simulink library "xpcmeasurementcomputinglib"  (Simulink 6.0)
settings: Solver=ode45  SolverMode=SingleTasking  StartTime=0.0  StopTime=10.0  RelTol=1e-3
undefined symbols (not defined in the file or in its folder): madcbciodas, madcbpcidas, madcbpcidas1600, mctr05checks, mdacbisa, mdacbpcidas, mdacbpcidas1600, mdacbpcidda0x12, mdiocbpcipdisox, menccbcioquadcount, misa8255, mpci8255, mtccb
libraries: xpcmeasurementcomputinglib x18
(part 2 of 4)

== system xpcmeasurementcomputinglib/D/A ==
  "CIO-DAC08 " : S-Function  InitFcn=mdacbisa(1);  FunctionName=dacbisa  Parameters=channel, range, reset, initValue, sampletime, baseaddress, boardType  mask(dacbisa){channel=[1], range=[-10], reset=[1], initValue=[0], sampletime=0.001, baseaddress=0x300}
      mask prompts: channel "Channel vector:"; range "Range vector:"; reset "Reset vector:"; initValue "Initial value vector:"; sampletime "Sample time:"; baseaddress "Base address (i.e. 0xd000):"
      mask help:
      | CIO-DAC08
      | ComputerBoards
      | Analog Output
      mask init:
      | baseaddress=hex2dec(baseaddress(3:end));
      | boardType=2;
      | [reset, initValue] = mdacbisa(2, channel, range, reset, initValue, baseaddress, boardType);
      mask Help: helpview(fullfile(docroot, 'mapfiles', 'xpc.map'), 'ComputerBoards_CIO-DAC08_DA')
      mask Display: disp('CIO-DAC08\nComputerBoards\nAnalog Output');port_label('input',1,'1');
  "CIO-DAC08 16 " : S-Function  InitFcn=mdacbisa(1);  FunctionName=dacbisa  Parameters=channel, range, reset, initValue, sampletime, baseaddress, boardType  mask(dacbisa){channel=[1], range=[-10], reset=[1], initValue=[0], sampletime=0.001, baseaddress=0x300}
      mask prompts: channel "Channel vector:"; range "Range vector:"; reset "Reset vector:"; initValue "Initial value vector:"; sampletime "Sample time:"; baseaddress "Base address (i.e. 0xd000):"
      mask help:
      | CIO-DAC08/16
      | ComputerBoards
      | Analog Output
      mask init:
      | baseaddress=hex2dec(baseaddress(3:end));
      | boardType=5;
      | [reset, initValue] = mdacbisa(2, channel, range, reset, initValue, baseaddress, boardType);
      mask Help: helpview(fullfile(docroot, 'mapfiles', 'xpc.map'), 'ComputerBoards_CIO-DAC08-16_DA')
      mask Display: disp('CIO-DAC08/16\nComputerBoards\nAnalog Output');port_label('input',1,'1');
  "CIO-DAC16 " : S-Function  InitFcn=mdacbisa(1);  FunctionName=dacbisa  Parameters=channel, range, reset, initValue, sampletime, baseaddress, boardType  mask(dacbisa){channel=[1], range=[-10], reset=[1], initValue=[0], sampletime=0.001, baseaddress=0x300}
      mask prompts: channel "Channel vector:"; range "Range vector:"; reset "Reset vector:"; initValue "Initial value vector:"; sampletime "Sample time:"; baseaddress "Base address (i.e. 0xd000):"
      mask help:
      | CIO-DAC16
      | ComputerBoards
      | Analog Output
      mask init:
      | baseaddress=hex2dec(baseaddress(3:end));
      | boardType=3;
      | [reset, initValue] = mdacbisa(2, channel, range, reset, initValue, baseaddress, boardType);
      mask Help: helpview(fullfile(docroot, 'mapfiles', 'xpc.map'), 'ComputerBoards_CIO-DAC16_DA')
      mask Display: disp('CIO-DAC16\nComputerBoards\nAnalog Output');port_label('input',1,'1');
  "CIO-DAC16 16 " : S-Function  InitFcn=mdacbisa(1);  FunctionName=dacbisa  Parameters=channel, range, reset, initValue, sampletime, baseaddress, boardType  mask(dacbisa){channel=[1], range=[-10], reset=[1], initValue=[0], sampletime=0.001, baseaddress=0x300}
      mask prompts: channel "Channel vector:"; range "Range vector:"; reset "Reset vector:"; initValue "Initial value vector:"; sampletime "Sample time:"; baseaddress "Base address (i.e. 0xd000):"
      mask help:
      | CIO-DAC16/16
      | ComputerBoards
      | Analog Output
      mask init:
      | baseaddress=hex2dec(baseaddress(3:end));
      | boardType=6;
      | [reset, initValue] = mdacbisa(2, channel, range, reset, initValue, baseaddress, boardType);
      mask Help: helpview(fullfile(docroot, 'mapfiles', 'xpc.map'), 'ComputerBoards_CIO-DAC16-16_DA')
      mask Display: disp('CIO-DAC16/16\nComputerBoards\nAnalog Output');port_label('input',1,'1');
  "CIO-DAS1601 12 " : S-Function  InitFcn=mdacbisa(1);  FunctionName=dacbisa  Parameters=channel, range, reset, initValue, sampletime, baseaddress, boardType  mask(dacbisa){channel=[1], range=[-10], reset=[1], initValue=[0], sampletime=0.001, baseaddress=0x300}
      mask prompts: channel "Channel vector:"; range "Range vector:"; reset "Reset vector:"; initValue "Initial value vector:"; sampletime "Sample time:"; baseaddress "Base address (i.e. 0xd000):"
      mask help:
      | CIO-DAS1601/12
      | ComputerBoards
      | Analog Output
      mask init:
      | baseaddress=hex2dec(baseaddress(3:end));
      | boardType=8;
      | [reset, initValue] = mdacbisa(2, channel, range, reset, initValue, baseaddress, boardType);
      mask Help: helpview(fullfile(docroot, 'mapfiles', 'xpc.map'), 'ComputerBoards_CIO-DAS1601-12_DA')
      mask Display: disp('CIO-DAS1601/12\nComputerBoards\nAnalog Output');port_label('input',1,'1');
  "CIO-DAS1602 12 " : S-Function  InitFcn=mdacbisa(1);  FunctionName=dacbisa  Parameters=channel, range, reset, initValue, sampletime, baseaddress, boardType  mask(dacbisa){channel=[1], range=[-10], reset=[1], initValue=[0], sampletime=0.001, baseaddress=0x300}
      mask prompts: channel "Channel vector:"; range "Range vector:"; reset "Reset vector:"; initValue "Initial value vector:"; sampletime "Sample time:"; baseaddress "Base address (i.e. 0xd000):"
      mask help:
      | CIO-DAS1602/12
      | ComputerBoards
      | Analog Output
      mask init:
      | baseaddress=hex2dec(baseaddress(3:end));
      | boardType=9;
      | [reset, initValue] = mdacbisa(2, channel, range, reset, initValue, baseaddress, boardType);
      mask Help: helpview(fullfile(docroot, 'mapfiles', 'xpc.map'), 'ComputerBoards_CIO-DAS1602-12_DA')
      mask Display: disp('CIO-DAS1602/12\nComputerBoards\nAnalog Output');port_label('input',1,'1');
  "CIO-DAS1602 16 " : S-Function  InitFcn=mdacbisa(1);  FunctionName=dacbisa  Parameters=channel, range, reset, initValue, sampletime, baseaddress, boardType  mask(dacbisa){channel=[1], range=[-10], reset=[1], initValue=[0], sampletime=0.001, baseaddress=0x300}
      mask prompts: channel "Channel vector:"; range "Range vector:"; reset "Reset vector:"; initValue "Initial value vector:"; sampletime "Sample time:"; baseaddress "Base address (i.e. 0xd000):"
      mask help:
      | CIO-DAS1602/16
      | ComputerBoards
      | Analog Output
      mask init:
      | baseaddress=hex2dec(baseaddress(3:end));
      | boardType=10;
      | [reset, initValue] = mdacbisa(2, channel, range, reset, initValue, baseaddress, boardType);
      mask Help: helpview(fullfile(docroot, 'mapfiles', 'xpc.map'), 'ComputerBoards_CIO-DAS1602-16_DA')
      mask Display: disp('CIO-DAS1602/16\nComputerBoards\nAnalog Output');port_label('input',1,'1');
  "CIO-DDA06 " : S-Function  InitFcn=mdacbisa(1);  FunctionName=dacbisa  Parameters=channel, range, reset, initValue, sampletime, baseaddress, boardType  mask(dacbisa){channel=[1], range=[-10], reset=[1], initValue=[0], sampletime=0.001, baseaddress=0x300}
      mask prompts: channel "Channel vector:"; range "Range vector:"; reset "Reset vector:"; initValue "Initial value vector:"; sampletime "Sample time:"; baseaddress "Base address (i.e. 0xd000):"
      mask help:
      | CIO-DDA06
      | ComputerBoards
      | Analog Output
      mask init:
      | baseaddress=hex2dec(baseaddress(3:end));
      | boardType=1;
      | [reset, initValue] = mdacbisa(2, channel, range, reset, initValue, baseaddress, boardType);
      mask Help: helpview(fullfile(docroot, 'mapfiles', 'xpc.map'), 'ComputerBoards_CIO-DDA06_DA')
      mask Display: disp('CIO-DDA06\nComputerBoards\nAnalog Output');port_label('input',1,'1');
  "CIO-DDA06 16 " : S-Function  InitFcn=mdacbisa(1);  FunctionName=dacbisa  Parameters=channel, range, reset, initValue, sampletime, baseaddress, boardType  mask(dacbisa){channel=[1], range=[-10], reset=[1], initValue=[0], sampletime=0.001, baseaddress=0x300}
      mask prompts: channel "Channel vector:"; range "Range vector:"; reset "Reset vector:"; initValue "Initial value vector:"; sampletime "Sample time:"; baseaddress "Base address (i.e. 0xd000):"
      mask help:
      | CIO-DDA06/16
      | ComputerBoards
      | Analog Output
      mask init:
      | baseaddress=hex2dec(baseaddress(3:end));
      | boardType=4;
      | [reset, initValue] = mdacbisa(2, channel, range, reset, initValue, baseaddress, boardType);
      mask Help: helpview(fullfile(docroot, 'mapfiles', 'xpc.map'), 'ComputerBoards_CIO-DDA06-16_DA')
      mask Display: disp('CIO-DDA06/16\nComputerBoards\nAnalog Output');port_label('input',1,'1');
  "PC104-DAC06 " : S-Function  InitFcn=mdacbisa(1);  FunctionName=dacbisa  Parameters=channel, range, reset, initValue, sampletime, baseaddress, boardType  mask(dacbisa){channel=[1], range=[-10], reset=[1], initValue=[0], sampletime=0.001, baseaddress=0x300}
      mask prompts: channel "Channel vector:"; range "Range vector:"; reset "Reset vector:"; initValue "Initial value vector:"; sampletime "Sample time:"; baseaddress "Base address (i.e. 0xd000):"
      mask help:
      | PC104-DAC06
      | ComputerBoards
      | Analog Output
      mask init:
      | baseaddress=hex2dec(baseaddress(3:end));
      | boardType=7;
      | [reset, initValue] = mdacbisa(2, channel, range, reset, initValue, baseaddress, boardType);
      mask Help: helpview(fullfile(docroot, 'mapfiles', 'xpc.map'), 'ComputerBoards_PC104-DAC06_DA')
      mask Display: disp('PC104-DAC06\nComputerBoards\nAnalog Output');port_label('input',1,'1');
  "PCI-DAS1200 " : S-Function  InitFcn=mdacbpcidas(1);  FunctionName=dacbpcidas  Parameters=channel, range, reset, initValue, sampletime, pci_dev, boardType  mask(dacbpcidda0x12){channel=[1], range=[-10], reset=[1], initValue=[0], sampletime=0.001, pci_dev=-1}
      mask prompts: channel "Channel vector:"; range "Range vector:"; reset "Reset vector:"; initValue "Initial value vector:"; sampletime "Sample time:"; pci_dev "PCI slot (-1: autosearch):"
      mask help:
      | PCI-DAS1200
      | ComputerBoards
      | Analog Output
      mask init:
      | boardType=1;
      | [reset, initValue] = mdacbpcidas(2,channel,range,pci_dev,boardType,reset,initValue);
      mask Help: helpview(fullfile(docroot, 'mapfiles', 'xpc.map'), 'ComputerBoards_PCI-DAS1200_DA')
      mask Display: disp('PCI-DAS1200\nComputerBoards\nAnalog Output');port_label('input',1,'1');
  "PCI-DAS1602 12 " : S-Function  InitFcn=mdacbpcidas1600(1);  FunctionName=dacbpcidas1600  Parameters=channel, range, reset, initValue, sampletime, pci_dev, boardType  mask(dacbpcidas160212){channel=[1], range=[-10], reset=[1], initValue=[0], sampletime=0.001, pci_dev=-1}
      mask prompts: channel "Channel vector:"; range "Range vector:"; reset "Reset vector:"; initValue "Initial value vector:"; sampletime "Sample time:"; pci_dev "PCI slot (-1: autosearch):"
      mask help:
      | PCI-DAS1602/12
      | ComputerBoards
      | Analog Output
      mask init:
      | boardType=1;
      | [range, reset, initValue] = mdacbpcidas1600(2,channel,range,pci_dev,boardType,reset,initValue);
      mask Help: helpview(fullfile(docroot, 'mapfiles', 'xpc.map'), 'ComputerBoards_PCI-DAS1602-12_DA')
      mask Display: disp('PCI-DAS1602/12\nComputerBoards\nAnalog Output');port_label('input',1,'1');
  "PCI-DAS1602 16 " : S-Function  InitFcn=mdacbpcidas1600(1);  FunctionName=dacbpcidas1600  Parameters=channel, range, reset, initValue, sampletime, pci_dev, boardType  mask(dacbpcidas160216){channel=[1], range=[-10], reset=[1], initValue=[0], sampletime=0.001, pci_dev=-1}
      mask prompts: channel "Channel vector:"; range "Range vector:"; reset "Reset vector:"; initValue "Initial value vector:"; sampletime "Sample time:"; pci_dev "PCI slot (-1: autosearch):"
      mask help:
      | PCI-DAS1602/16
      | ComputerBoards
      | Analog Output
      mask init:
      | boardType=2;
      | [range, reset, initValue] = mdacbpcidas1600(2,channel,range,pci_dev,boardType,reset,initValue);
      mask Help: helpview(fullfile(docroot, 'mapfiles', 'xpc.map'), 'ComputerBoards_PCI-DAS1602-16_DA')
      mask Display: disp('PCI-DAS1602/16\nComputerBoards\nAnalog Output');port_label('input',1,'1');
  "PCI-DDA02 12 " : S-Function  InitFcn=mdacbpcidda0x12(1);  FunctionName=dacbpcidda0x12  Parameters=channel, range, reset, initValue, sampletime,pci_dev,boardType  mask(dacbpcidda0x12){channel=[1], range=[-10], reset=[1], initValue=[0], sampletime=0.001, pci_dev=-1}
      mask prompts: channel "Channel vector:"; range "Range vector:"; reset "Reset vector:"; initValue "Initial value vector:"; sampletime "Sample time:"; pci_dev "PCI slot (-1: autosearch):"
      mask help:
      | PCI-DDA02/12
      | ComputerBoards
      | Analog Output
      mask init:
      | boardType=1;
      | [reset, initValue] = mdacbpcidda0x12(2,channel,range,reset,initValue,pci_dev,boardType);
      mask Help: helpview(fullfile(docroot, 'mapfiles', 'xpc.map'), 'ComputerBoards_PCI-DDA02-12_DA')
      mask Display: disp('PCI-DDA02/12\nComputerBoards\nAnalog Output');port_label('input',1,'1');
  "PCI-DDA02 16 " : S-Function  InitFcn=mdacbpcidda0x12(1);  FunctionName=dacbpcidda0x12  Parameters=channel, range, reset, initValue, sampletime,pci_dev,boardType  mask(dacbpcidda0x16){channel=[1], range=[-10], reset=[1], initValue=[0], sampletime=0.001, pci_dev=-1}
      mask prompts: channel "Channel vector:"; range "Range vector:"; reset "Reset vector:"; initValue "Initial value vector:"; sampletime "Sample time:"; pci_dev "PCI slot (-1: autosearch):"
      mask help:
      | PCI-DDA02/16
      | ComputerBoards
      | Analog Output
      mask init:
      | boardType=4;
      | [reset, initValue] = mdacbpcidda0x12(2,channel,range,reset,initValue,pci_dev,boardType);
      mask Help: helpview(fullfile(docroot, 'mapfiles', 'xpc.map'), 'ComputerBoards_PCI-DDA02-16_DA')
      mask Display: disp('PCI-DDA02/16\nComputerBoards\nAnalog Output');port_label('input',1,'1');
  "PCI-DDA04 12 " : S-Function  InitFcn=mdacbpcidda0x12(1);  FunctionName=dacbpcidda0x12  Parameters=channel, range, reset, initValue, sampletime,pci_dev,boardType  mask(dacbpcidda0x12){channel=[1], range=[-10], reset=[1], initValue=[0], sampletime=0.001, pci_dev=-1}
      mask prompts: channel "Channel vector:"; range "Range vector:"; reset "Reset vector:"; initValue "Initial value vector:"; sampletime "Sample time:"; pci_dev "PCI slot (-1: autosearch):"
      mask help:
      | PCI-DDA04/12
      | ComputerBoards
      | Analog Output
      mask init:
      | boardType=2;
      | [reset, initValue] = mdacbpcidda0x12(2,channel,range,reset,initValue,pci_dev,boardType);
      mask Help: helpview(fullfile(docroot, 'mapfiles', 'xpc.map'), 'ComputerBoards_PCI-DDA04-12_DA')
      mask Display: disp('PCI-DDA04/12\nComputerBoards\nAnalog Output');port_label('input',1,'1');
  "PCI-DDA04 16 " : S-Function  InitFcn=mdacbpcidda0x12(1);  FunctionName=dacbpcidda0x12  Parameters=channel, range, reset, initValue, sampletime,pci_dev,boardType  mask(dacbpcidda0x16){channel=[1], range=[-10], reset=[1], initValue=[0], sampletime=0.001, pci_dev=-1}
      mask prompts: channel "Channel vector:"; range "Range vector:"; reset "Reset vector:"; initValue "Initial value vector:"; sampletime "Sample time:"; pci_dev "PCI slot (-1: autosearch):"
      mask help:
      | PCI-DDA04/16
      | ComputerBoards
      | Analog Output
      mask init:
      | boardType=5;
      | [reset, initValue] = mdacbpcidda0x12(2,channel,range,reset,initValue,pci_dev,boardType);
      mask Help: helpview(fullfile(docroot, 'mapfiles', 'xpc.map'), 'ComputerBoards_PCI-DDA04-16_DA')
      mask Display: disp('PCI-DDA04/16\nComputerBoards\nAnalog Output');port_label('input',1,'1');
  "PCI-DDA08 12 " : S-Function  InitFcn=mdacbpcidda0x12(1);  FunctionName=dacbpcidda0x12  Parameters=channel, range, reset, initValue, sampletime,pci_dev,boardType  mask(dacbpcidda0x12){channel=[1], range=[-10], reset=[1], initValue=[0], sampletime=0.001, pci_dev=-1}
      mask prompts: channel "Channel vector:"; range "Range vector:"; reset "Reset vector:"; initValue "Initial value vector:"; sampletime "Sample time:"; pci_dev "PCI slot (-1: autosearch):"
      mask help:
      | PCI-DDA08/12
      | ComputerBoards
      | Analog Output
      mask init:
      | boardType=3;
      | [reset, initValue] = mdacbpcidda0x12(2,channel,range,reset,initValue,pci_dev,boardType);
      mask Help: helpview(fullfile(docroot, 'mapfiles', 'xpc.map'), 'ComputerBoards_PCI-DDA08-12_DA')
      mask Display: disp('PCI-DDA08/12\nComputerBoards\nAnalog Output');port_label('input',1,'1');
  "PCI-DDA08 16 " : S-Function  InitFcn=mdacbpcidda0x12(1);  FunctionName=dacbpcidda0x12  Parameters=channel, range, reset, initValue, sampletime,pci_dev,boardType  mask(dacbpcidda0x16){channel=[1], range=[-10], reset=[1], initValue=[0], sampletime=0.001, pci_dev=-1}
      mask prompts: channel "Channel vector:"; range "Range vector:"; reset "Reset vector:"; initValue "Initial value vector:"; sampletime "Sample time:"; pci_dev "PCI slot (-1: autosearch):"
      mask help:
      | PCI-DDA08/16
      | ComputerBoards
      | Analog Output
      mask init:
      | boardType=6;
      | [reset, initValue] = mdacbpcidda0x12(2,channel,range,reset,initValue,pci_dev,boardType);
      mask Help: helpview(fullfile(docroot, 'mapfiles', 'xpc.map'), 'ComputerBoards_PCI-DDA08-16_DA')
      mask Display: disp('PCI-DDA08/16\nComputerBoards\nAnalog Output');port_label('input',1,'1');
  "PCIM-DAS1602 16 " : S-Function  InitFcn=mdacbpcidda0x12(1);  FunctionName=dacbpcidda0x12  Parameters=channel, range, reset, initValue, sampletime,pci_dev,boardType  mask(dacbpcidda0x12){channel=[1], range=[-10], reset=[1], initValue=[0], sampletime=0.001, pci_dev=-1}
      mask prompts: channel "Channel vector:"; range "Range vector:"; reset "Reset vector:"; initValue "Initial value vector:"; sampletime "Sample time:"; pci_dev "PCI slot (-1: autosearch):"
      mask help:
      | PCIM-DAS1602/16
      | ComputerBoards
      | Analog Output
      mask init:
      | boardType=8;
      | [reset, initValue] = mdacbpcidda0x12(2,channel,range,reset,initValue,pci_dev,boardType);
      mask Help: helpview(fullfile(docroot, 'mapfiles', 'xpc.map'), 'ComputerBoards_PCIM-DAS1602-16_DA')
      mask Display: disp('PCIM-DAS1602/16\nComputerBoards\nAnalog Output');port_label('input',1,'1');
  "PCIM-DDA06 16 " : S-Function  InitFcn=mdacbpcidda0x12(1);  FunctionName=dacbpcidda0x12  Parameters=channel, range, reset, initValue, sampletime,pci_dev,boardType  mask(dacbpcidda0x12){channel=[1], range=[-10], reset=[1], initValue=[0], sampletime=0.001, pci_dev=-1}
      mask prompts: channel "Channel vector:"; range "Range vector:"; reset "Reset vector:"; initValue "Initial value vector:"; sampletime "Sample time:"; pci_dev "PCI slot (-1: autosearch):"
      mask help:
      | PCIM-DDA06/16
      | ComputerBoards
      | Analog Output
      mask init:
      | boardType=7;
      | [reset, initValue] = mdacbpcidda0x12(2,channel,range,reset,initValue,pci_dev,boardType);
      mask Help: helpview(fullfile(docroot, 'mapfiles', 'xpc.map'), 'ComputerBoards_PCIM-DDA06-16_DA')
      mask Display: disp('PCIM-DDA06/16\nComputerBoards\nAnalog Output');port_label('input',1,'1');

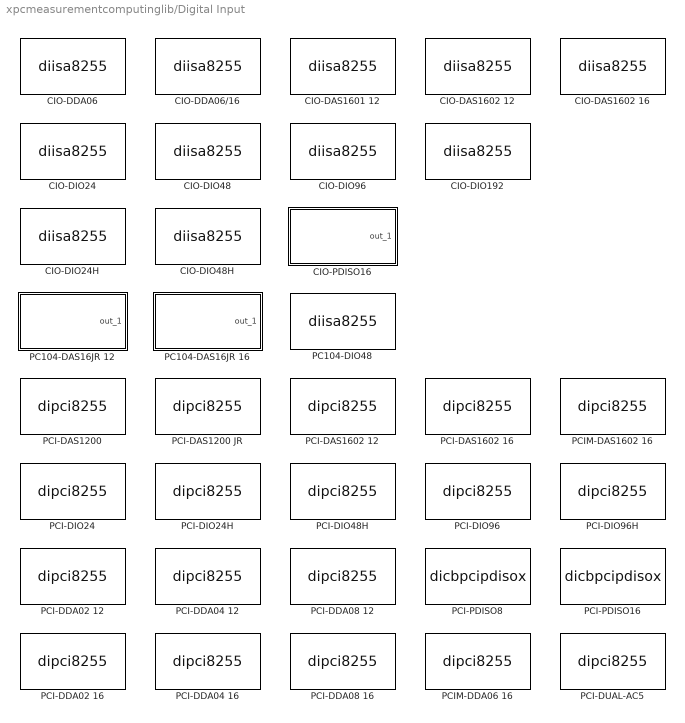
== system xpcmeasurementcomputinglib/Digital Input ==
  "CIO-DAS1601 12 " : S-Function  InitFcn=misa8255(1);  FunctionName=diisa8255  Parameters=channel, port, sampletime, baseaddress, control  mask(dicbciodas160112){channel=[1], port=A, chip=1, sampletime=0.001, baseaddress=0x300}
      mask prompts: channel "Channel vector:"; sampletime "Sample time:"; baseaddress "Base address (i.e. 0xd000):"
      mask help:
      | CIO-DAS1601/12
      | ComputerBoards
      | Digital Input
      mask init:
      | baseaddress=hex2dec(baseaddress(3:end));
      | control=155;
      | [baseaddress,control, maskdisplay, maskdescription]=misa8255(2, chip, port, channel, baseaddress);
      | set_param(gcb, 'MaskDisplay', maskdisplay);
      | set_param(gcb, 'MaskDescription', maskdescription);
      mask Help: helpview(fullfile(docroot, 'mapfiles', 'xpc.map'), 'ComputerBoards_CIO-DAS1601-12_DIN')
      mask StyleString: edit,popup(A|B|C),popup(1),edit,edit
      mask Display: disp('CIO-DAS1601/12\nComputerBoards\nDigital Input');port_label('output',1,'1');
  "CIO-DAS1602 12 " : S-Function  InitFcn=misa8255(1);  FunctionName=diisa8255  Parameters=channel, port, sampletime, baseaddress, control  mask(dicbciodas160212){channel=[1], port=A, chip=1, sampletime=0.001, baseaddress=0x300}
      mask prompts: channel "Channel vector:"; sampletime "Sample time:"; baseaddress "Base address (i.e. 0xd000):"
      mask help:
      | CIO-DAS1602/12
      | ComputerBoards
      | Digital Input
      mask init: same as xpcmeasurementcomputinglib/Digital Input/CIO-DAS1601 12 
      mask Help: helpview(fullfile(docroot, 'mapfiles', 'xpc.map'), 'ComputerBoards_CIO-DAS1602-12_DIN')
      mask StyleString: edit,popup(A|B|C),popup(1),edit,edit
      mask Display: disp('CIO-DAS1602/12\nComputerBoards\nDigital Input');port_label('output',1,'1');
  "CIO-DAS1602 16 " : S-Function  InitFcn=misa8255(1);  FunctionName=diisa8255  Parameters=channel, port, sampletime, baseaddress, control  mask(dicbciodas160216){channel=[1], port=A, chip=1, sampletime=0.001, baseaddress=0x300}
      mask prompts: channel "Channel vector:"; sampletime "Sample time:"; baseaddress "Base address (i.e. 0xd000):"
      mask help:
      | CIO-DAS1602/16
      | ComputerBoards
      | Digital Input
      mask init: same as xpcmeasurementcomputinglib/Digital Input/CIO-DAS1601 12 
      mask Help: helpview(fullfile(docroot, 'mapfiles', 'xpc.map'), 'ComputerBoards_CIO-DAS1602-16_DIN')
      mask StyleString: edit,popup(A|B|C),popup(1),edit,edit
      mask Display: disp('CIO-DAS1602/16\nComputerBoards\nDigital Input');port_label('output',1,'1');
  "CIO-DDA06 " : S-Function  InitFcn=misa8255(1);  FunctionName=diisa8255  Parameters=channel, port, sampletime, baseaddress, control  mask(dicbciodda06){channel=[1], port=A, chip=1, sampletime=0.001, baseaddress=0x300}
      mask prompts: channel "Channel vector:"; sampletime "Sample time:"; baseaddress "Base address (i.e. 0xd000):"
      mask help:
      | CIO-DDA06
      | ComputerBoards
      | Digital Input
      mask init: same as xpcmeasurementcomputinglib/Digital Input/CIO-DAS1601 12 
      mask Help: helpview(fullfile(docroot, 'mapfiles', 'xpc.map'), 'ComputerBoards_CIO-DDA06_DIN')
      mask StyleString: edit,popup(A|B|C),popup(1),edit,edit
      mask Display: disp('CIO-DDA06\nComputerBoards\nDigital Input');port_label('output',1,'1');
  "CIO-DDA06/16 " : S-Function  InitFcn=misa8255(1);  FunctionName=diisa8255  Parameters=channel, port, sampletime, baseaddress, control  mask(dicbciodda0616){channel=[1], port=A, chip=1, sampletime=0.001, baseaddress=0x300}
      mask prompts: channel "Channel vector:"; sampletime "Sample time:"; baseaddress "Base address (i.e. 0xd000):"
      mask help:
      | CIO-DDA06/16
      | ComputerBoards
      | Digital Input
      mask init: same as xpcmeasurementcomputinglib/Digital Input/CIO-DAS1601 12 
      mask Help: helpview(fullfile(docroot, 'mapfiles', 'xpc.map'), 'ComputerBoards_CIO-DDA06-16_DIN')
      mask StyleString: edit,popup(A|B|C),popup(1),edit,edit
      mask Display: disp('CIO-DDA06/16\nComputerBoards\nDigital Input');port_label('output',1,'1');
  "CIO-DIO192 " : S-Function  InitFcn=misa8255(1);  FunctionName=diisa8255  Parameters=channel, port, sampletime, baseaddress, control  mask(dicbciodio192){channel=[1], port=A, chip=1, sampletime=0.001, baseaddress=0x300}
      mask prompts: channel "Channel vector:"; sampletime "Sample time:"; baseaddress "Base address (i.e. 0xd000):"
      mask help:
      | CIO-DIO192
      | ComputerBoards
      | Digital Input
      mask init: same as xpcmeasurementcomputinglib/Digital Input/CIO-DAS1601 12 
      mask Help: helpview(fullfile(docroot, 'mapfiles', 'xpc.map'), 'ComputerBoards_CIO-DIO192_DIN')
      mask StyleString: edit,popup(A|B|C),popup(1|2|3|4|5|6|7|8),edit,edit
      mask Display: disp('CIO-DIO192\nComputerBoards\nDigital Input');port_label('output',1,'1');
  "CIO-DIO24 " : S-Function  InitFcn=misa8255(1);  FunctionName=diisa8255  Parameters=channel, port, sampletime, baseaddress, control  mask(dicbciodio24){channel=[1], port=A, chip=1, sampletime=0.001, baseaddress=0x300}
      mask prompts: channel "Channel vector:"; sampletime "Sample time:"; baseaddress "Base address (i.e. 0xd000):"
      mask help:
      | CIO-DIO24
      | ComputerBoards
      | Digital Input
      mask init: same as xpcmeasurementcomputinglib/Digital Input/CIO-DAS1601 12 
      mask Help: helpview(fullfile(docroot, 'mapfiles', 'xpc.map'), 'ComputerBoards_CIO-DIO24_DIN')
      mask StyleString: edit,popup(A|B|C),popup(1),edit,edit
      mask Display: disp('CIO-DIO24\nComputerBoards\nDigital Input');port_label('output',1,'1');
  "CIO-DIO24H " : S-Function  InitFcn=misa8255(1);  FunctionName=diisa8255  Parameters=channel, port, sampletime, baseaddress, control  mask(dicbciodio24h){channel=[1], port=A, chip=1, sampletime=0.001, baseaddress=0x300}
      mask prompts: channel "Channel vector:"; sampletime "Sample time:"; baseaddress "Base address (i.e. 0xd000):"
      mask help:
      | CIO-DIO24H
      | ComputerBoards
      | Digital Input
      mask init: same as xpcmeasurementcomputinglib/Digital Input/CIO-DAS1601 12 
      mask Help: helpview(fullfile(docroot, 'mapfiles', 'xpc.map'), 'ComputerBoards_CIO-DIO24H_DIN')
      mask StyleString: edit,popup(A|B|C),popup(1),edit,edit
      mask Display: disp('CIO-DIO24H\nComputerBoards\nDigital Input');port_label('output',1,'1');
  "CIO-DIO48 " : S-Function  InitFcn=misa8255(1);  FunctionName=diisa8255  Parameters=channel, port, sampletime, baseaddress, control  mask(dicbciodio48){channel=[1], port=A, chip=1, sampletime=0.001, baseaddress=0x300}
      mask prompts: channel "Channel vector:"; sampletime "Sample time:"; baseaddress "Base address (i.e. 0xd000):"
      mask help:
      | CIO-DIO48
      | ComputerBoards
      | Digital Input
      mask init: same as xpcmeasurementcomputinglib/Digital Input/CIO-DAS1601 12 
      mask Help: helpview(fullfile(docroot, 'mapfiles', 'xpc.map'), 'ComputerBoards_CIO-DIO48_DIN')
      mask StyleString: edit,popup(A|B|C),popup(1|2),edit,edit
      mask Display: disp('CIO-DIO48\nComputerBoards\nDigital Input');port_label('output',1,'1');
  "CIO-DIO48H " : S-Function  InitFcn=misa8255(1);  FunctionName=diisa8255  Parameters=channel, port, sampletime, baseaddress, control  mask(dicbciodio48h){channel=[1], port=A, chip=1, sampletime=0.001, baseaddress=0x300}
      mask prompts: channel "Channel vector:"; sampletime "Sample time:"; baseaddress "Base address (i.e. 0xd000):"
      mask help:
      | CIO-DIO48H
      | ComputerBoards
      | Digital Input
      mask init: same as xpcmeasurementcomputinglib/Digital Input/CIO-DAS1601 12 
      mask Help: helpview(fullfile(docroot, 'mapfiles', 'xpc.map'), 'ComputerBoards_CIO-DIO48H_DIN')
      mask StyleString: edit,popup(A|B|C),popup(1|2),edit,edit
      mask Display: disp('CIO-DIO48H\nComputerBoards\nDigital Input');port_label('output',1,'1');
  "CIO-DIO96 " : S-Function  InitFcn=misa8255(1);  FunctionName=diisa8255  Parameters=channel, port, sampletime, baseaddress, control  mask(dicbciodio96){channel=[1], port=A, chip=1, sampletime=0.001, baseaddress=0x300}
      mask prompts: channel "Channel vector:"; sampletime "Sample time:"; baseaddress "Base address (i.e. 0xd000):"
      mask help:
      | CIO-DIO96
      | ComputerBoards
      | Digital Input
      mask init: same as xpcmeasurementcomputinglib/Digital Input/CIO-DAS1601 12 
      mask Help: helpview(fullfile(docroot, 'mapfiles', 'xpc.map'), 'ComputerBoards_CIO-DIO96_DIN')
      mask StyleString: edit,popup(A|B|C),popup(1|2|3|4),edit,edit
      mask Display: disp('CIO-DIO96\nComputerBoards\nDigital Input');port_label('output',1,'1');
  "CIO-PDISO16 " : Subsystem  EnableExecutionContextPropagation=on  mask(Digital Input Module){n_channels=1, port=1 (nearest to backplate), sample_time=0.001, baseaddress=0x300}
      mask prompts: n_channels "Number of channels:"; port "Section (connector):"; sample_time "Sample time:"; baseaddress "Base address (i.e. 0xd000):"
      mask help:
      | Computer Boards
      | CIO-PDISO16
      | Digital Input
      mask init:
      | baseaddress=hex2dec(baseaddress(3:end));
      mask Help: helpview(fullfile(docroot, 'mapfiles', 'xpc.map'), 'ComputerBoards_CIO-PDISO16_DIN')
      mask StyleString: edit,popup(1 (nearest to backplate)|2 (farthest from backplate)),edit,edit
      mask Display: disp('CIO-PDISO16\nComputerBoards\nDigital Input')
  "PC104-DAS16JR 12 " : Subsystem  EnableExecutionContextPropagation=on  mask(Digital Input Module){n_channels=1, sample_time=0.001, baseaddress=0x300}
      mask prompts: n_channels "Number of channels:"; sample_time "Sample time:"; baseaddress "Base address (i.e. 0xd000):"
      mask help:
      | Computer Boards
      | PC104-DAS16JR/12
      | Digital Input
      mask init:
      | baseaddress=hex2dec(baseaddress(3:end));
      mask Help: helpview(fullfile(docroot, 'mapfiles', 'xpc.map'), 'ComputerBoards_PC104-DAS16JR-12_DIN')
      mask Display: disp('PC104-DAS16JR/12\nComputerBoards\nDigital Input')
  "PC104-DAS16JR 16 " : Subsystem  EnableExecutionContextPropagation=on  mask(Digital Input Module){n_channels=1, sample_time=0.001, baseaddress=0x300}
      mask prompts: n_channels "Number of channels:"; sample_time "Sample time:"; baseaddress "Base address (i.e. 0xd000):"
      mask help:
      | Computer Boards
      | PC104-DAS16JR/16
      | Digital Input
      mask init:
      | baseaddress=hex2dec(baseaddress(3:end));
      mask Help: helpview(fullfile(docroot, 'mapfiles', 'xpc.map'), 'ComputerBoards_PC104-DAS16JR-16_DIN')
      mask Display: disp('PC104-DAS16JR/16\nComputerBoards\nDigital Input')
  "PC104-DIO48 " : S-Function  InitFcn=misa8255(1);  FunctionName=diisa8255  Parameters=channel, port, sampletime, baseaddress, control  mask(dicbpc104dio48){channel=[1], port=A, chip=1, sampletime=0.001, baseaddress=0x300}
      mask prompts: channel "Channel vector:"; sampletime "Sample time:"; baseaddress "Base address (i.e. 0xd000):"
      mask help:
      | PC104-DIO48
      | ComputerBoards
      | Digital Input
      mask init: same as xpcmeasurementcomputinglib/Digital Input/CIO-DAS1601 12 
      mask Help: helpview(fullfile(docroot, 'mapfiles', 'xpc.map'), 'ComputerBoards_PC104-DIO48_DIN')
      mask StyleString: edit,popup(A|B|C),popup(1|2),edit,edit
      mask Display: disp('PC104-DIO48\nComputerBoards\nDigital Input');port_label('output',1,'1');
  "PCI-DAS1200 " : S-Function  InitFcn=mpci8255(1);  FunctionName=dipci8255  Parameters=channel, port, chip, sampletime, slot, control, boardType  mask(dicbpcidas1200){channel=[1], port=A, chip=1, sampletime=0.001, slot=-1}
      mask prompts: channel "Channel vector:"; sampletime "Sample time:"; slot "PCI slot (-1: autosearch):"
      mask help:
      | PCI-DAS1200
      | ComputerBoards
      | Digital Input
      mask init:
      | control=155;
      | [boardType,control,maskdisplay,maskdescription]=mpci8255(2, chip, port, channel, slot);
      | set_param(gcb, 'MaskDisplay', maskdisplay);
      | set_param(gcb, 'MaskDescription', maskdescription);
      mask Help: helpview(fullfile(docroot, 'mapfiles', 'xpc.map'), 'ComputerBoards_PCI-DAS1200_DIN')
      mask StyleString: edit,popup(A|B|C),popup(1),edit,edit
      mask Display: disp('PCI-DAS1200\nComputerBoards\nDigital Input');port_label('output',1,'1');
  "PCI-DAS1200 JR " : S-Function  InitFcn=mpci8255(1);  FunctionName=dipci8255  Parameters=channel, port, chip, sampletime, slot, control, boardType  mask(dicbpcidas1200jr){channel=[1], port=A, chip=1, sampletime=0.001, slot=-1}
      mask prompts: channel "Channel vector:"; sampletime "Sample time:"; slot "PCI slot (-1: autosearch):"
      mask help:
      | PCI-DAS1200/JR
      | ComputerBoards
      | Digital Input
      mask init:
      | control=155;
      | [boardType,control,maskdisplay,maskdescription]=mpci8255(2, chip, port, channel, slot);
      | set_param(gcb, 'MaskDisplay', maskdisplay);
      | set_param(gcb, 'MaskDescription', maskdescription);
      mask Help: helpview(fullfile(docroot, 'mapfiles', 'xpc.map'), 'ComputerBoards_PCI-DAS1200-JR_DIN')
      mask StyleString: edit,popup(A|B|C),popup(1),edit,edit
      mask Display: disp('PCI-DAS1200/JR\nComputerBoards\nDigital Input');port_label('output',1,'1');
  "PCI-DAS1602 12 " : S-Function  InitFcn=mpci8255(1);  FunctionName=dipci8255  Parameters=channel, port, chip, sampletime, slot, control, boardType  mask(dicbpcidas160212){channel=[1], port=A, chip=1, sampletime=0.001, slot=-1}
      mask prompts: channel "Channel vector:"; sampletime "Sample time:"; slot "PCI slot (-1: autosearch):"
      mask help:
      | PCI-DAS1602/12
      | ComputerBoards
      | Digital Input
      mask init:
      | control=155;
      | [boardType,control,maskdisplay,maskdescription]=mpci8255(2, chip, port, channel, slot);
      | set_param(gcb, 'MaskDisplay', maskdisplay);
      | set_param(gcb, 'MaskDescription', maskdescription);
      mask Help: helpview(fullfile(docroot, 'mapfiles', 'xpc.map'), 'ComputerBoards_PCI-DAS1602-12_DIN')
      mask StyleString: edit,popup(A|B|C),popup(1),edit,edit
      mask Display: disp('PCI-DAS1602/12\nComputerBoards\nDigital Input');port_label('output',1,'1');
  "PCI-DAS1602 16 " : S-Function  InitFcn=mpci8255(1);  FunctionName=dipci8255  Parameters=channel, port, chip, sampletime, slot, control, boardType  mask(dicbpcidas160216){channel=[1], port=A, chip=1, sampletime=0.001, slot=-1}
      mask prompts: channel "Channel vector:"; sampletime "Sample time:"; slot "PCI slot (-1: autosearch):"
      mask help:
      | PCI-DAS1602/16
      | ComputerBoards
      | Digital Input
      mask init:
      | control=155;
      | [boardType,control,maskdisplay,maskdescription]=mpci8255(2, chip, port, channel, slot);
      | set_param(gcb, 'MaskDisplay', maskdisplay);
      | set_param(gcb, 'MaskDescription', maskdescription);
      mask Help: helpview(fullfile(docroot, 'mapfiles', 'xpc.map'), 'ComputerBoards_PCI-DAS1602-16_DIN')
      mask StyleString: edit,popup(A|B|C),popup(1),edit,edit
      mask Display: disp('PCI-DAS1602/16\nComputerBoards\nDigital Input');port_label('output',1,'1');
  "PCI-DDA02 12 " : S-Function  InitFcn=mpci8255(1);  FunctionName=dipci8255  Parameters=channel, port, chip, sampletime, slot, control, boardType  mask(dicbpcidda0212){channel=[1], port=A, chip=1, sampletime=0.001, slot=-1}
      mask prompts: channel "Channel vector:"; sampletime "Sample time:"; slot "PCI slot (-1: autosearch):"
      mask help:
      | PCI-DDA02/12
      | ComputerBoards
      | Digital Input
      mask init:
      | control=155;
      | [boardType,control,maskdisplay,maskdescription]=mpci8255(2, chip, port, channel, slot);
      | set_param(gcb, 'MaskDisplay', maskdisplay);
      | set_param(gcb, 'MaskDescription', maskdescription);
      mask Help: helpview(fullfile(docroot, 'mapfiles', 'xpc.map'), 'ComputerBoards_PCI-DDA02-12_DIN')
      mask StyleString: edit,popup(A|B|C),popup(1|2),edit,edit
      mask Display: disp('PCI-DDA02/12\nComputerBoards\nDigital Input');port_label('output',1,'1');
  "PCI-DDA02 16 " : S-Function  InitFcn=mpci8255(1);  FunctionName=dipci8255  Parameters=channel, port, chip, sampletime, slot, control, boardType  mask(dicbpcidda0216){channel=[1], port=A, chip=1, sampletime=0.001, slot=-1}
      mask prompts: channel "Channel vector:"; sampletime "Sample time:"; slot "PCI slot (-1: autosearch):"
      mask help:
      | PCI-DDA02/16
      | ComputerBoards
      | Digital Input
      mask init:
      | control=155;
      | [boardType,control,maskdisplay,maskdescription]=mpci8255(2, chip, port, channel, slot);
      | set_param(gcb, 'MaskDisplay', maskdisplay);
      | set_param(gcb, 'MaskDescription', maskdescription);
      mask Help: helpview(fullfile(docroot, 'mapfiles', 'xpc.map'), 'ComputerBoards_PCI-DDA02-16_DIN')
      mask StyleString: edit,popup(A|B|C),popup(1|2),edit,edit
      mask Display: disp('PCI-DDA02/16\nComputerBoards\nDigital Input');port_label('output',1,'1');
  "PCI-DDA04 12 " : S-Function  InitFcn=mpci8255(1);  FunctionName=dipci8255  Parameters=channel, port, chip, sampletime, slot, control, boardType  mask(dicbpcidda0412){channel=[1], port=A, chip=1, sampletime=0.001, slot=-1}
      mask prompts: channel "Channel vector:"; sampletime "Sample time:"; slot "PCI slot (-1: autosearch):"
      mask help:
      | PCI-DDA04/12
      | ComputerBoards
      | Digital Input
      mask init:
      | control=155;
      | [boardType,control,maskdisplay,maskdescription]=mpci8255(2, chip, port, channel, slot);
      | set_param(gcb, 'MaskDisplay', maskdisplay);
      | set_param(gcb, 'MaskDescription', maskdescription);
      mask Help: helpview(fullfile(docroot, 'mapfiles', 'xpc.map'), 'ComputerBoards_PCI-DDA04-12_DIN')
      mask StyleString: edit,popup(A|B|C),popup(1|2),edit,edit
      mask Display: disp('PCI-DDA04/12\nComputerBoards\nDigital Input');port_label('output',1,'1');
  "PCI-DDA04 16 " : S-Function  InitFcn=mpci8255(1);  FunctionName=dipci8255  Parameters=channel, port, chip, sampletime, slot, control, boardType  mask(dicbpcidda0416){channel=[1], port=A, chip=1, sampletime=0.001, slot=-1}
      mask prompts: channel "Channel vector:"; sampletime "Sample time:"; slot "PCI slot (-1: autosearch):"
      mask help:
      | PCI-DDA04/16
      | ComputerBoards
      | Digital Input
      mask init:
      | control=155;
      | [boardType,control,maskdisplay,maskdescription]=mpci8255(2, chip, port, channel, slot);
      | set_param(gcb, 'MaskDisplay', maskdisplay);
      | set_param(gcb, 'MaskDescription', maskdescription);
      mask Help: helpview(fullfile(docroot, 'mapfiles', 'xpc.map'), 'ComputerBoards_PCI-DDA04-16_DIN')
      mask StyleString: edit,popup(A|B|C),popup(1|2),edit,edit
      mask Display: disp('PCI-DDA04/16\nComputerBoards\nDigital Input');port_label('output',1,'1');
  "PCI-DDA08 12 " : S-Function  InitFcn=mpci8255(1);  FunctionName=dipci8255  Parameters=channel, port, chip, sampletime, slot, control, boardType  mask(dicbpcidda0812){channel=[1], port=A, chip=1, sampletime=0.001, slot=-1}
      mask prompts: channel "Channel vector:"; sampletime "Sample time:"; slot "PCI slot (-1: autosearch):"
      mask help:
      | PCI-DDA08/12
      | ComputerBoards
      | Digital Input
      mask init:
      | control=155;
      | [boardType,control,maskdisplay,maskdescription]=mpci8255(2, chip, port, channel, slot);
      | set_param(gcb, 'MaskDisplay', maskdisplay);
      | set_param(gcb, 'MaskDescription', maskdescription);
      mask Help: helpview(fullfile(docroot, 'mapfiles', 'xpc.map'), 'ComputerBoards_PCI-DDA08-12_DIN')
      mask StyleString: edit,popup(A|B|C),popup(1|2),edit,edit
      mask Display: disp('PCI-DDA08/12\nComputerBoards\nDigital Input');port_label('output',1,'1');
  "PCI-DDA08 16 " : S-Function  InitFcn=mpci8255(1);  FunctionName=dipci8255  Parameters=channel, port, chip, sampletime, slot, control, boardType  mask(dicbpcidda0816){channel=[1], port=A, chip=1, sampletime=0.001, slot=-1}
      mask prompts: channel "Channel vector:"; sampletime "Sample time:"; slot "PCI slot (-1: autosearch):"
      mask help:
      | PCI-DDA08/16
      | ComputerBoards
      | Digital Input
      mask init:
      | control=155;
      | [boardType,control,maskdisplay,maskdescription]=mpci8255(2, chip, port, channel, slot);
      | set_param(gcb, 'MaskDisplay', maskdisplay);
      | set_param(gcb, 'MaskDescription', maskdescription);
      mask Help: helpview(fullfile(docroot, 'mapfiles', 'xpc.map'), 'ComputerBoards_PCI-DDA08-16_DIN')
      mask StyleString: edit,popup(A|B|C),popup(1|2),edit,edit
      mask Display: disp('PCI-DDA08/16\nComputerBoards\nDigital Input');port_label('output',1,'1');
  "PCI-DIO24 " : S-Function  InitFcn=mpci8255(1);  FunctionName=dipci8255  Parameters=channel, port, chip, sampletime, slot, control, boardType  mask(dicbpcidio24){channel=[1], port=A, chip=1, sampletime=0.001, slot=-1}
      mask prompts: channel "Channel vector:"; sampletime "Sample time:"; slot "PCI slot (-1: autosearch):"
      mask help:
      | PCI-DIO24
      | ComputerBoards
      | Digital Input
      mask init:
      | control=155;
      | [boardType,control,maskdisplay,maskdescription]=mpci8255(2, chip, port, channel, slot);
      | set_param(gcb, 'MaskDisplay', maskdisplay);
      | set_param(gcb, 'MaskDescription', maskdescription);
      mask Help: helpview(fullfile(docroot, 'mapfiles', 'xpc.map'), 'ComputerBoards_PCI-DIO24_DIN')
      mask StyleString: edit,popup(A|B|C),popup(1),edit,edit
      mask Display: disp('PCI-DIO24\nComputerBoards\nDigital Input');port_label('output',1,'1');
  "PCI-DIO24H " : S-Function  InitFcn=mpci8255(1);  FunctionName=dipci8255  Parameters=channel, port, chip, sampletime, slot, control, boardType  mask(dicbpcidio24h){channel=[1], port=A, chip=1, sampletime=0.001, slot=-1}
      mask prompts: channel "Channel vector:"; sampletime "Sample time:"; slot "PCI slot (-1: autosearch):"
      mask help:
      | PCI-DIO24H
      | ComputerBoards
      | Digital Input
      mask init:
      | control=155;
      | [boardType,control,maskdisplay,maskdescription]=mpci8255(2, chip, port, channel, slot);
      | set_param(gcb, 'MaskDisplay', maskdisplay);
      | set_param(gcb, 'MaskDescription', maskdescription);
      mask Help: helpview(fullfile(docroot, 'mapfiles', 'xpc.map'), 'ComputerBoards_PCI-DIO24H_DIN')
      mask StyleString: edit,popup(A|B|C),popup(1),edit,edit
      mask Display: disp('PCI-DIO24H\nComputerBoards\nDigital Input');port_label('output',1,'1');
  "PCI-DIO48H " : S-Function  InitFcn=mpci8255(1);  FunctionName=dipci8255  Parameters=channel, port, chip, sampletime, slot, control, boardType  mask(dicbpcidio48h){channel=[1], port=A, chip=1, sampletime=0.001, slot=-1}
      mask prompts: channel "Channel vector:"; sampletime "Sample time:"; slot "PCI slot (-1: autosearch):"
      mask help:
      | PCI-DIO48H
      | ComputerBoards
      | Digital Input
      mask init:
      | control=155;
      | [boardType,control,maskdisplay,maskdescription]=mpci8255(2, chip, port, channel, slot);
      | set_param(gcb, 'MaskDisplay', maskdisplay);
      | set_param(gcb, 'MaskDescription', maskdescription);
      mask Help: helpview(fullfile(docroot, 'mapfiles', 'xpc.map'), 'ComputerBoards_PCI-DIO48H_DIN')
      mask StyleString: edit,popup(A|B|C),popup(1|2),edit,edit
      mask Display: disp('PCI-DIO48H\nComputerBoards\nDigital Input');port_label('output',1,'1');
  "PCI-DIO96 " : S-Function  InitFcn=mpci8255(1);  FunctionName=dipci8255  Parameters=channel, port, chip, sampletime, slot, control, boardType  mask(dicbpcidio96){channel=[1], port=A, chip=1, sampletime=0.001, slot=-1}
      mask prompts: channel "Channel vector:"; sampletime "Sample time:"; slot "PCI slot (-1: autosearch):"
      mask help:
      | PCI-DIO96
      | ComputerBoards
      | Digital Input
      mask init:
      | control=155;
      | [boardType,control,maskdisplay,maskdescription]=mpci8255(2, chip, port, channel, slot);
      | set_param(gcb, 'MaskDisplay', maskdisplay);
      | set_param(gcb, 'MaskDescription', maskdescription);
      mask Help: helpview(fullfile(docroot, 'mapfiles', 'xpc.map'), 'ComputerBoards_PCI-DIO96_DIN')
      mask StyleString: edit,popup(A|B|C),popup(1|2|3|4),edit,edit
      mask Display: disp('PCI-DIO96\nComputerBoards\nDigital Input');port_label('output',1,'1');
  "PCI-DIO96H " : S-Function  InitFcn=mpci8255(1);  FunctionName=dipci8255  Parameters=channel, port, chip, sampletime, slot, control, boardType  mask(dicbpcidio96h){channel=[1], port=A, chip=1, sampletime=0.001, slot=-1}
      mask prompts: channel "Channel vector:"; sampletime "Sample time:"; slot "PCI slot (-1: autosearch):"
      mask help:
      | PCI-DIO96H
      | ComputerBoards
      | Digital Input
      mask init:
      | control=155;
      | [boardType,control,maskdisplay,maskdescription]=mpci8255(2, chip, port, channel, slot);
      | set_param(gcb, 'MaskDisplay', maskdisplay);
      | set_param(gcb, 'MaskDescription', maskdescription);
      mask Help: helpview(fullfile(docroot, 'mapfiles', 'xpc.map'), 'ComputerBoards_PCI-DIO96H_DIN')
      mask StyleString: edit,popup(A|B|C),popup(1|2|3|4),edit,edit
      mask Display: disp('PCI-DIO96H\nComputerBoards\nDigital Input');port_label('output',1,'1');
  "PCI-DUAL-AC5 " : S-Function  InitFcn=mpci8255(1);  FunctionName=dipci8255  Parameters=channel, port, chip, sampletime, slot, control, boardType  mask(dicbpcidualac5){channel=[1], port=A, chip=1, sampletime=0.001, slot=-1}
      mask prompts: channel "Channel vector:"; sampletime "Sample time:"; slot "PCI slot (-1: autosearch):"
      mask help:
      | PCI-DUAL-AC5
      | ComputerBoards
      | Digital Input
      mask init:
      | control=155;
      | [boardType,control,maskdisplay,maskdescription]=mpci8255(2, chip, port, channel, slot);
      | set_param(gcb, 'MaskDisplay', maskdisplay);
      | set_param(gcb, 'MaskDescription', maskdescription);
      mask Help: helpview(fullfile(docroot, 'mapfiles', 'xpc.map'), 'ComputerBoards_PCI-DUAL-AC5_DIN')
      mask StyleString: edit,popup(A|B|C),popup(1|2|3|4),edit,edit
      mask Display: disp('PCI-DUAL-AC5\nComputerBoards\nDigital Input');port_label('output',1,'1');
  "PCI-PDISO16 " : S-Function  InitFcn=mdiocbpcipdisox(1);  FunctionName=dicbpcipdisox  Parameters=channel, port, sampletime, slot, filter, boardType  mask(dicbpcipdiso16){channel=[1], filter=[0], port=A, sampletime=0.001, slot=-1}
      mask prompts: channel "Channel vector:"; filter "Filter vector:"; sampletime "Sample time:"; slot "PCI slot (-1: autosearch):"
      mask help:
      | PCI-DISO16
      | ComputerBoards
      | Digital Input
      mask init:
      | [boardType,filter,maskdisplay,maskdescription]=mdiocbpcipdisox(2, port, channel, filter, slot);
      | set_param(gcb, 'MaskDisplay', maskdisplay);
      | set_param(gcb, 'MaskDescription', maskdescription);
      mask Help: helpview(fullfile(docroot, 'mapfiles', 'xpc.map'), 'ComputerBoards_PCI-PDISO16_DIN')
      mask StyleString: edit,edit,popup(A|B),edit,edit
      mask Display: disp('PCI-DISO16\nComputerBoards\nDigital Input');port_label('output',1,'1');
  "PCI-PDISO8 " : S-Function  InitFcn=mdiocbpcipdisox(1);  FunctionName=dicbpcipdisox  Parameters=channel, port, sampletime, slot, filter, boardType  mask(dicbpcipdiso8){channel=[1], filter=[0], port=A, sampletime=0.001, slot=-1}
      mask prompts: channel "Channel vector:"; filter "Filter vector:"; sampletime "Sample time:"; slot "PCI slot (-1: autosearch):"
      mask help:
      | PCI-DISO8
      | ComputerBoards
      | Digital Input
      mask init:
      | [boardType,filter,maskdisplay,maskdescription]=mdiocbpcipdisox(2, port, channel, filter, slot);
      | set_param(gcb, 'MaskDisplay', maskdisplay);
      | set_param(gcb, 'MaskDescription', maskdescription);
      mask Help: helpview(fullfile(docroot, 'mapfiles', 'xpc.map'), 'ComputerBoards_PCI-PDISO8_DIN')
      mask StyleString: edit,edit,popup(A|B),edit,edit
      mask Display: disp('PCI-DISO8\nComputerBoards\nDigital Input');port_label('output',1,'1');
  "PCIM-DAS1602 16 " : S-Function  InitFcn=mpci8255(1);  FunctionName=dipci8255  Parameters=channel, port, chip, sampletime, slot, control, boardType  mask(dicbpcimdas160216){channel=[1], port=A, chip=1, sampletime=0.001, slot=-1}
      mask prompts: channel "Channel vector:"; sampletime "Sample time:"; slot "PCI slot (-1: autosearch):"
      mask help:
      | PCIM-DAS1602/16
      | ComputerBoards
      | Digital Input
      mask init:
      | control=155;
      | [boardType,control,maskdisplay,maskdescription]=mpci8255(2, chip, port, channel, slot);
      | set_param(gcb, 'MaskDisplay', maskdisplay);
      | set_param(gcb, 'MaskDescription', maskdescription);
      mask Help: helpview(fullfile(docroot, 'mapfiles', 'xpc.map'), 'ComputerBoards_PCIM-DAS1602-16_DIN')
      mask StyleString: edit,popup(A|B|C),popup(1),edit,edit
      mask Display: disp('PCIM-DAS1602/16\nComputerBoards\nDigital Input');port_label('output',1,'1');
  "PCIM-DDA06 16 " : S-Function  InitFcn=mpci8255(1);  FunctionName=dipci8255  Parameters=channel, port, chip, sampletime, slot, control, boardType  mask(dicbpcimdda0616){channel=[1], port=A, chip=1, sampletime=0.001, slot=-1}
      mask prompts: channel "Channel vector:"; sampletime "Sample time:"; slot "PCI slot (-1: autosearch):"
      mask help:
      | PCIM-DDA06/16
      | ComputerBoards
      | Digital Input
      mask init:
      | control=155;
      | [boardType,control,maskdisplay,maskdescription]=mpci8255(2, chip, port, channel, slot);
      | set_param(gcb, 'MaskDisplay', maskdisplay);
      | set_param(gcb, 'MaskDescription', maskdescription);
      mask Help: helpview(fullfile(docroot, 'mapfiles', 'xpc.map'), 'ComputerBoards_PCIM-DDA06-16_DIN')
      mask StyleString: edit,popup(A|B|C),popup(1),edit,edit
      mask Display: disp('PCIM-DDA06/16\nComputerBoards\nDigital Input');port_label('output',1,'1');
